simulink model "onuncu_yontem"  (R2023a)
settings: Solver=VariableStepAuto  StartTime=0.0  StopTime=10.0  RelTol=1e-3
settings Model: Creator=Lenovo  LastModifiedBy=Lenovo

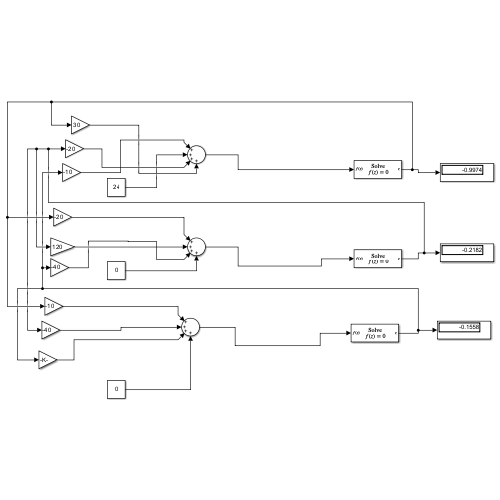
[thumbnail: Simulink's stored preview of the top-level diagram]
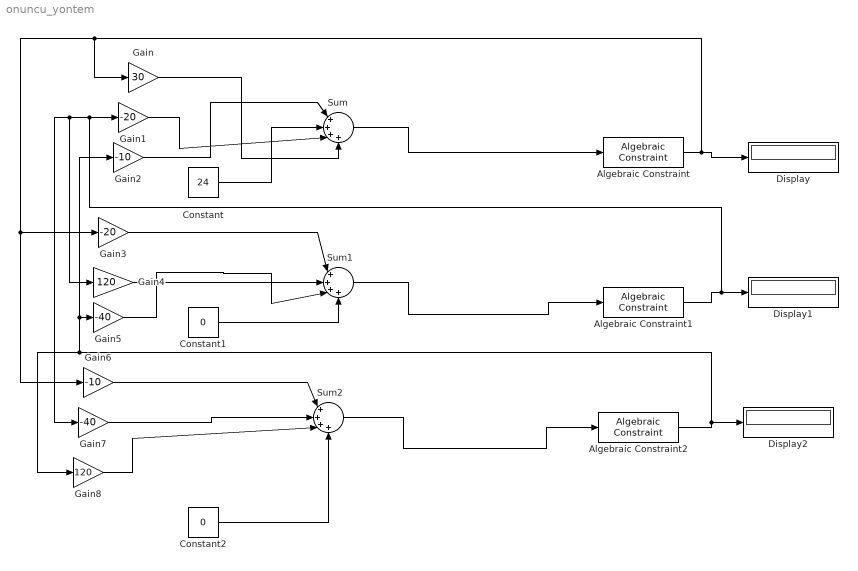
== system onuncu_yontem ==
  Algebraic Constraint : AlgebraicConstraint
  Algebraic Constraint1 : AlgebraicConstraint
  Algebraic Constraint2 : AlgebraicConstraint
  Constant : Constant  Value=24
  Constant1 : Constant  Value=0
  Constant2 : Constant  Value=0
  Display : Display
  Display1 : Display
  Display2 : Display
  Gain : Gain  Gain=30
  Gain1 : Gain  Gain=-20
  Gain2 : Gain  Gain=-10
  Gain3 : Gain  Gain=-20
  Gain4 : Gain  Gain=120
  Gain5 : Gain  Gain=-40
  Gain6 : Gain  Gain=-10
  Gain7 : Gain  Gain=-40
  Gain8 : Gain  Gain=120
  Sum : Sum  Inputs=|++++
  Sum1 : Sum  Inputs=|++++
  Sum2 : Sum  Inputs=|++++
  wires:
  Algebraic Constraint1/1 -> Gain1/1, Gain7/1, Gain4/1, Display1/1
  Algebraic Constraint2/1 -> Gain8/1, Gain5/1, Gain2/1, Display2/1
  Constant/1 -> Sum/2
  Gain2/1 -> Sum/1
  Gain1/1 -> Sum/3
  Gain/1 -> Sum/4
  Sum/1 -> Algebraic Constraint/1
  Gain3/1 -> Sum1/1
  Gain4/1 -> Sum1/2
  Gain5/1 -> Sum1/3
  Constant1/1 -> Sum1/4
  Gain6/1 -> Sum2/1
  Gain7/1 -> Sum2/2
  Gain8/1 -> Sum2/3
  Constant2/1 -> Sum2/4
  Sum1/1 -> Algebraic Constraint1/1
  Sum2/1 -> Algebraic Constraint2/1
  Algebraic Constraint/1 -> Gain6/1, Gain3/1, Gain/1, Display/1
